simulink model "VerificaLMI"  (R2025b)
settings: Solver=VariableStepAuto  StartTime=0.0  StopTime=15.0  RelTol=1e-3
values from neighbouring files (symbols this model uses):
  A = double(subs(A_sym, p_eq_instabile, val_instabili))    [SvolgimentoEsame.m]
  B = double(subs(B_sym, p_eq_instabile, val_instabili))    [SvolgimentoEsame.m]
  C = eye(4)    [SvolgimentoEsame.m]
  D = zeros(4, 1)    [SvolgimentoEsame.m]
  K_3 = Nval / Qval    [SvolgimentoEsame.m]
  X_initial = [x0; dx0; th0; dth0]    [SvolgimentoEsame.m]
  X_ref = [x_ref_val; 0; 0; 0]    [SvolgimentoEsame.m]
settings Model: Creator=salvo  LastModifiedBy=salvo

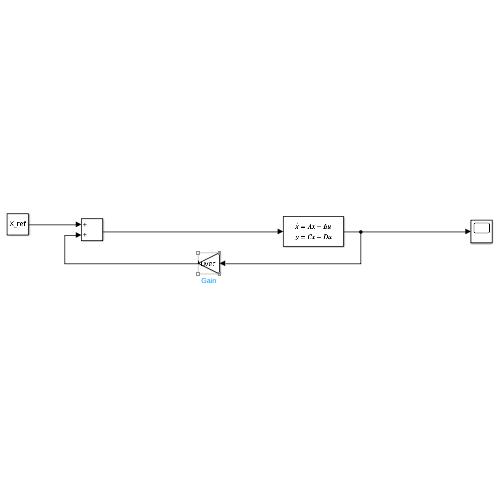
[thumbnail: Simulink's stored preview of the top-level diagram]
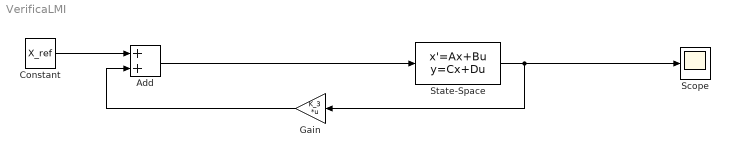
== system VerificaLMI ==
  Add : Sum
  Constant : Constant  Value=X_ref
  Gain : Gain  Gain=K_3  Multiplication=Matrix(K*u) (u vector)
  Scope : Scope
      settings: ActiveDisplayYMinimum=-13.921095644631857  ActiveDisplayYMaximum=9.6824002013036345
  State-Space : StateSpace  A=A  B=B  C=C  D=D  InitialCondition=X_initial
  wires:
  Constant/1 -> Add/1
  State-Space/1 -> Gain/1, Scope/1
  Gain/1 -> Add/2
  Add/1 -> State-Space/1
